simulink model "InsertedCoinsFcn"  (R2019b)
settings: Solver=FixedStepAuto  StartTime=0.0  StopTime=Inf  FixedStep=SAMPLING_TIME  RelTol=1e-3
undefined symbols (not defined in the file): INSERTED_COINS_REGISTER, INTEGER_000_CENTS, INTEGER_010_CENTS, INTEGER_020_CENTS, INTEGER_050_CENTS, INTEGER_100_CENTS, INTEGER_200_CENTS, SAMPLING_TIME
libraries: Components x9
Description:
  | % Copyright 2019 The MathWorks, Inc.
settings Model: DataDictionary=Parameters.sldd  EnableAccessToBaseWorkspace=off  EnablePacing=on  Creator=sdupertu  LastModifiedBy=sdupertu
settings DataIOCC: SaveOutput=off  SaveTime=off
settings OptimizationCC: DefaultParameterBehavior=Inlined  EnhancedBackFolding=on  PassReuseOutputArgsAs=Individual arguments  OptimizeBlockOrder=speed  DifferentSizesBufferReuse=on  OptimizationCustomize=off  EfficientTunableParamExpr=on
settings DebuggingCC: ParameterTunabilityLossMsg=error  PregeneratedLibrarySubsystemCodeDiagnostic=none  ArithmeticOperatorsInVariantConditions=warning
settings ModelReferenceCC: EnableParallelModelReferenceBuilds=on
settings SFSimCC: SimUseLocalCustomCode=off  MATLABDynamicMemAlloc=off  CustomCodeUndefinedFunction=UseInterfaceOnly
settings RTWCC: SystemTargetFile=ert.tlc  TemplateMakefile=ert_default_tmf  GenerateReport=on  RTWUseLocalCustomCode=off  IncludeHyperlinkInReport=on  LaunchReport=on  GenerateTraceInfo=on  GenerateTraceReport=on  GenerateTraceReportSl=on  GenerateTraceReportSf=on  GenerateTraceReportEml=on  GenerateWebview=on  GenerateCodeMetricsReport=on
settings CodeAppCC: ForceParamTrailComments=on  IgnoreCustomStorageClasses=off  MaxIdLength=61  OperatorAnnotations=on  SimulinkDataObjDesc=on  SFDataObjDesc=on  InsertBlockDesc=on
settings ERTTargetCC: TargetLangStandard=C99 (ISO)  GenerateSampleERTMain=on  InlinedParameterPlacement=NonHierarchical  ERTCustomFileTemplate=example_file_process.tlc

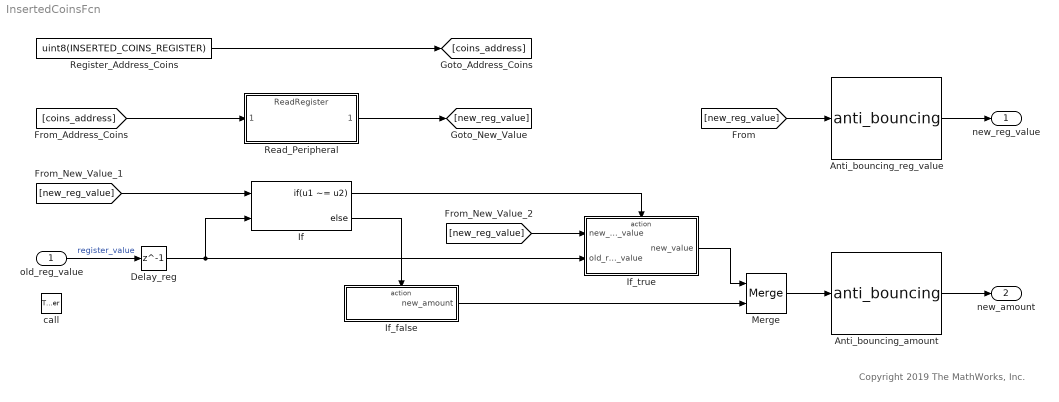
== system InsertedCoinsFcn ==
  note: Copyright 2019 The MathWorks, Inc.
  old_reg_value : Inport  OutDataTypeStr=uint8  PortDimensions=1
  call : TriggerPort  TriggerType=either  VariantControl=Variant  PortDimensions=1  TriggerSignalSampleTime=[SAMPLING_TIME,0]
  Anti_bouncing_amount : Components/anti_bouncing  SystemSampleTime=-1  Latency=0  AutoFrameSizeCalculation=off
  Anti_bouncing_reg_value : Components/anti_bouncing  SystemSampleTime=-1  Latency=0  AutoFrameSizeCalculation=off
  Delay_reg : Delay  DelayLength=1  InitialCondition=0
  If : If  NumInputs=2  IfExpression=u1 ~= u2
  If_false : Subsystem  TreatAsAtomicUnit=on
  If_true : Subsystem  TreatAsAtomicUnit=on
  Merge : Merge
  Read_Peripheral : ModelReference  ModelNameDialog=ReadRegister  SimulationMode=Normal  ModelReferenceVersion=1.124
  Register_Address_Coins : Constant  Value=uint8(INSERTED_COINS_REGISTER)  SampleTime=-1
  new_reg_value : Outport  OutDataTypeStr=uint8  PortDimensions=1  VectorParamsAs1DForOutWhenUnconnected=off
  new_amount : Outport  Port=2  OutDataTypeStr=uint8  PortDimensions=1  VectorParamsAs1DForOutWhenUnconnected=off
  wires:
  Register_Address_Coins/1 -> [coins_address]
  [coins_address] -> Read_Peripheral/1
  Read_Peripheral/1 -> [new_reg_value]
  If/2 -> If_false/Action
  If_true/1(new_value) -> Merge/1
  [new_reg_value] -> If/1
  If_false/1(new_amount) -> Merge/2
  If/1 -> If_true/Action
  [new_reg_value] -> If_true/1(new_reg_value)
  old_reg_value/1 -> Delay_reg/1  "register_value"
  Delay_reg/1 -> If/2, If_true/2(old_reg_value)
  Merge/1 -> Anti_bouncing_amount/1
  Anti_bouncing_amount/1 -> new_amount/1
  [new_reg_value] -> Anti_bouncing_reg_value/1
  Anti_bouncing_reg_value/1 -> new_reg_value/1

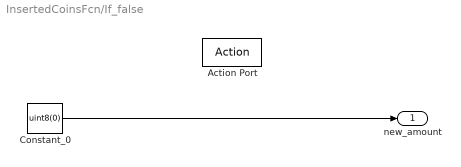
== system InsertedCoinsFcn/If_false ==
  Action Port : ActionPort  ActionPortLabel=else
  Constant_0 : Constant  Value=uint8(0)  SampleTime=-1
  new_amount : Outport  InitialOutput=0  VectorParamsAs1DForOutWhenUnconnected=off
  wires:
  Constant_0/1 -> new_amount/1

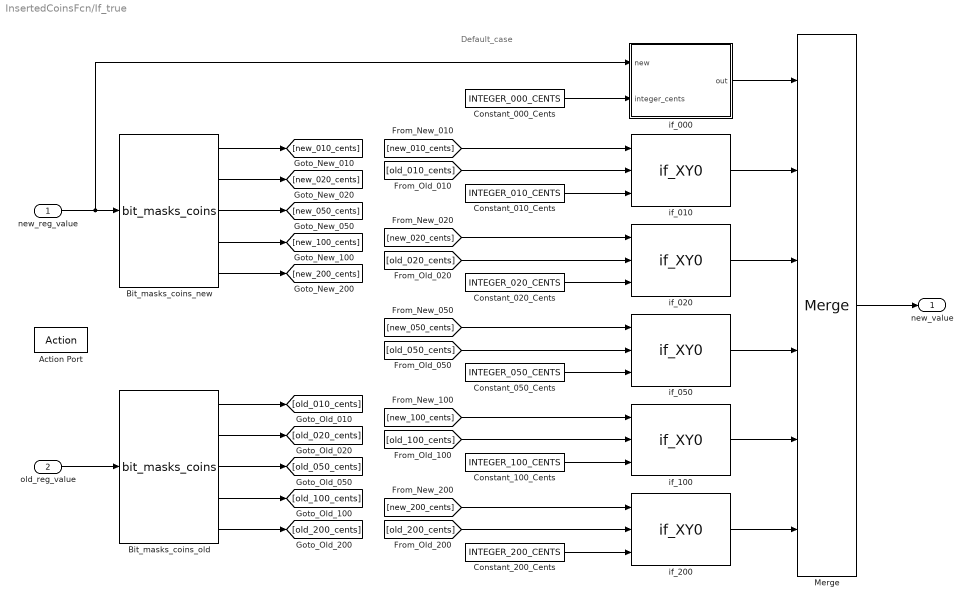
== system InsertedCoinsFcn/If_true ==
  note: Default_case
  new_reg_value : Inport
  old_reg_value : Inport  Port=2
  Action Port : ActionPort  ActionPortLabel=if(u1 ~= u2)
  Bit_masks_coins_new : Components/bit_masks_coins  SystemSampleTime=-1  Latency=0  AutoFrameSizeCalculation=off
  Bit_masks_coins_old : Components/bit_masks_coins  SystemSampleTime=-1  Latency=0  AutoFrameSizeCalculation=off
  Constant_000_Cents : Constant  Value=INTEGER_000_CENTS  SampleTime=-1
  Constant_010_Cents : Constant  Value=INTEGER_010_CENTS  SampleTime=-1
  Constant_020_Cents : Constant  Value=INTEGER_020_CENTS  SampleTime=-1
  Constant_050_Cents : Constant  Value=INTEGER_050_CENTS  SampleTime=-1
  Constant_100_Cents : Constant  Value=INTEGER_100_CENTS  SampleTime=-1
  Constant_200_Cents : Constant  Value=INTEGER_200_CENTS  SampleTime=-1
  Merge : Merge  Inputs=6
  if_000 : Subsystem
  if_010 : Components/if_XY0  SystemSampleTime=-1  Latency=0  AutoFrameSizeCalculation=off
  if_020 : Components/if_XY0  SystemSampleTime=-1  Latency=0  AutoFrameSizeCalculation=off
  if_050 : Components/if_XY0  SystemSampleTime=-1  Latency=0  AutoFrameSizeCalculation=off
  if_100 : Components/if_XY0  SystemSampleTime=-1  Latency=0  AutoFrameSizeCalculation=off
  if_200 : Components/if_XY0  SystemSampleTime=-1  Latency=0  AutoFrameSizeCalculation=off
  new_value : Outport  VectorParamsAs1DForOutWhenUnconnected=off
  wires:
  Constant_000_Cents/1 -> if_000/2(integer_cents)
  if_000/1(out) -> Merge/1
  Constant_200_Cents/1 -> if_200/3
  Constant_100_Cents/1 -> if_100/3
  Constant_050_Cents/1 -> if_050/3
  Constant_020_Cents/1 -> if_020/3
  Constant_010_Cents/1 -> if_010/3
  if_010/1 -> Merge/2
  [old_010_cents] -> if_010/2
  [new_010_cents] -> if_010/1
  Bit_masks_coins_new/5 -> [new_200_cents]
  Bit_masks_coins_old/5 -> [old_200_cents]
  [old_200_cents] -> if_200/2
  if_200/1 -> Merge/6
  [new_200_cents] -> if_200/1
  Merge/1 -> new_value/1
  if_100/1 -> Merge/5
  if_020/1 -> Merge/3
  if_050/1 -> Merge/4
  [old_100_cents] -> if_100/2
  [new_100_cents] -> if_100/1
  [old_050_cents] -> if_050/2
  [new_050_cents] -> if_050/1
  [old_020_cents] -> if_020/2
  [new_020_cents] -> if_020/1
  Bit_masks_coins_old/2 -> [old_020_cents]
  Bit_masks_coins_old/3 -> [old_050_cents]
  Bit_masks_coins_old/4 -> [old_100_cents]
  Bit_masks_coins_old/1 -> [old_010_cents]
  Bit_masks_coins_new/3 -> [new_050_cents]
  Bit_masks_coins_new/4 -> [new_100_cents]
  Bit_masks_coins_new/2 -> [new_020_cents]
  Bit_masks_coins_new/1 -> [new_010_cents]
  old_reg_value/1 -> Bit_masks_coins_old/1
  new_reg_value/1 -> Bit_masks_coins_new/1, if_000/1(new)

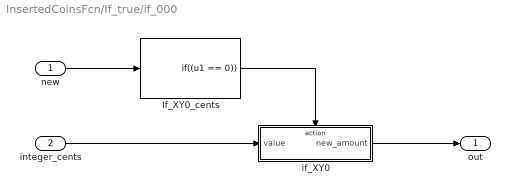
== system InsertedCoinsFcn/If_true/if_000 ==
  new : Inport
  integer_cents : Inport  Port=2
  If_XY0_cents : If  IfExpression=(u1 == 0)  ShowElse=off
  if_XY0 : Subsystem  TreatAsAtomicUnit=on
  out : Outport  VectorParamsAs1DForOutWhenUnconnected=off
  wires:
  if_XY0/1(new_amount) -> out/1
  If_XY0_cents/1 -> if_XY0/Action
  new/1 -> If_XY0_cents/1
  integer_cents/1 -> if_XY0/1(value)

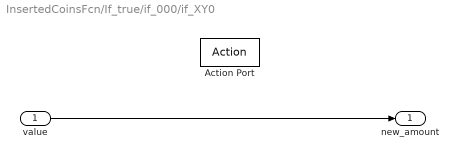
== system InsertedCoinsFcn/If_true/if_000/if_XY0 ==
  value : Inport
  Action Port : ActionPort  ActionPortLabel=if((u1 == 0))
  new_amount : Outport  VectorParamsAs1DForOutWhenUnconnected=off
  wires:
  value/1 -> new_amount/1
